simulink model "firstpart"  (R2022a)
settings: Solver=FixedStepAuto  StartTime=0.0  StopTime=5  FixedStep=0.25  RelTol=1e-3
settings Model: Creator=P1oruN7  LastModifiedBy=P1oruN7

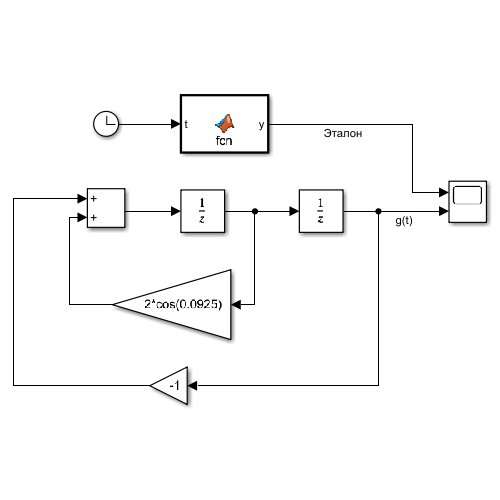
[thumbnail: Simulink's stored preview of the top-level diagram]
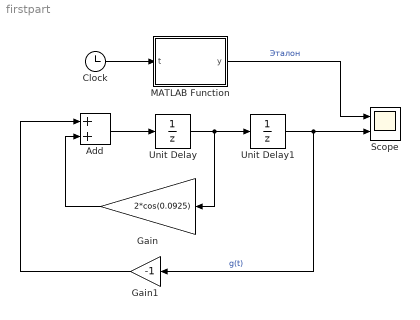
== system firstpart ==
  Add : Sum
  Clock : Clock
  Gain : Gain  Gain=2*cos(0.0925)
  Gain1 : Gain  Gain=-1
  MATLAB Function : MATLAB Function  TreatAsAtomicUnit=on
  Scope : Scope  NumInputPorts=2
  Unit Delay : UnitDelay  InitialCondition=1.3*sin(0.0925)  SampleTime=-1  HasFrameUpgradeWarning=on
  Unit Delay1 : UnitDelay  SampleTime=-1  HasFrameUpgradeWarning=on
  wires:
  Unit Delay/1 -> Gain/1, Unit Delay1/1
  Unit Delay1/1 -> Scope/2, Gain1/1  "g(t)"
  Add/1 -> Unit Delay/1
  Gain/1 -> Add/2
  Gain1/1 -> Add/1
  Clock/1 -> MATLAB Function/1(t)
  MATLAB Function/1(y) -> Scope/1  "Эталон"

== matlab function firstpart/MATLAB Function ==
  data: t input; y output
function y = fcn(t)

y = 1.3*sin(0.37*t);
